simulink model "lqr_simulink"  (R2014b)
settings: Solver=ode45  StartTime=0.0  StopTime=1  RelTol=1e-3
values from neighbouring files (symbols this model uses):
  Bm = 0.0    (= 0)    [base.m]    (also in base_parameter.m; lqr_parameter.m; pid_perameter.m)
  Jm = 24.5*10^-7    (= 2.45e-06)    [base.m]    (also in base_parameter.m = 1.08e-06; lqr_parameter.m = 1.08e-06; pid_perameter.m)
  Ke = 173*0.10472    (= 18.11656)    [base.m]    (also in base_parameter.m = 0.0234050839587; lqr_parameter.m = 0.0234050839587; pid_perameter.m = 173)
  Kt = 55.2*10^-3    (= 0.0552)    [base.m]    (also in base_parameter.m = 0.00285; lqr_parameter.m = 0.00285; pid_perameter.m)
  La = 5.02*10^-3    (= 0.00502)    [base.m]    (also in base_parameter.m = 0.000238; lqr_parameter.m = 0.000238; pid_perameter.m)
  Ra = 40    [base.m]    (also in base_parameter.m = 2.32; lqr_parameter.m = 2.32; pid_perameter.m)
undefined symbols (not defined in the file or in its folder): K
settings Model: Creator=Admin  LastModifiedBy=nghia

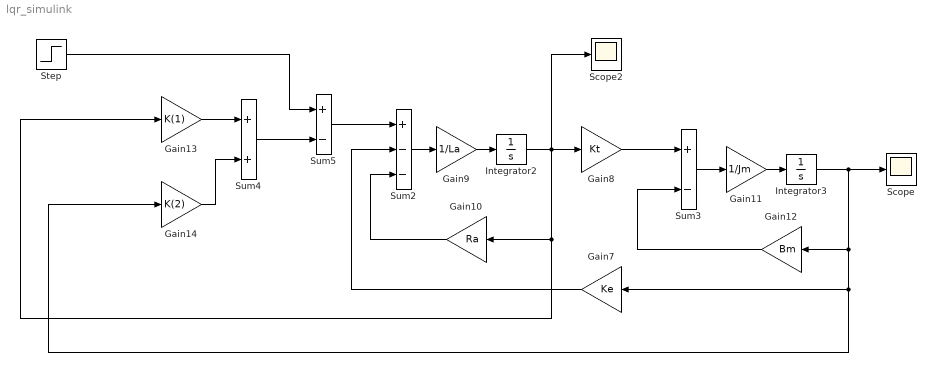
== system lqr_simulink ==
  Gain10 : Gain  Gain=Ra
  Gain11 : Gain  Gain=1/Jm
  Gain12 : Gain  Gain=Bm
  Gain13 : Gain  Gain=K(1)
  Gain14 : Gain  Gain=K(2)
  Gain7 : Gain  Gain=Ke
  Gain8 : Gain  Gain=Kt
  Gain9 : Gain  Gain=1/La
  Integrator2 : Integrator
  Integrator3 : Integrator
  Scope : Scope
      settings: YMin=0  YMax=10
  Scope2 : Scope
      settings: YMin=0  YMax=10  SaveName=ScopeData2
  Step : Step  Time=0.1  SampleTime=0
  Sum2 : Sum  Inputs=+--
  Sum3 : Sum  Inputs=+-
  Sum4 : Sum
  Sum5 : Sum  Inputs=+-
  wires:
  Step/1 -> Sum5/1
  Gain7/1 -> Sum2/2
  Sum2/1 -> Gain9/1
  Gain9/1 -> Integrator2/1
  Gain10/1 -> Sum2/3
  Gain8/1 -> Sum3/1
  Sum3/1 -> Gain11/1
  Gain11/1 -> Integrator3/1
  Gain12/1 -> Sum3/2
  Gain13/1 -> Sum4/1
  Gain14/1 -> Sum4/2
  Sum4/1 -> Sum5/2
  Sum5/1 -> Sum2/1
  Integrator3/1 -> Scope/1, Gain14/1, Gain7/1, Gain12/1
  Integrator2/1 -> Gain13/1, Gain10/1, Scope2/1, Gain8/1
